simulink model "ps_mass_balance"  (R2025a)
settings: Solver=VariableStepAuto  StartTime=0.0  StopTime=10.0  RelTol=1e-3
libraries: nesl_utility x10, fl_lib x3
settings Model: Creator=degoede  LastModifiedBy=degoede

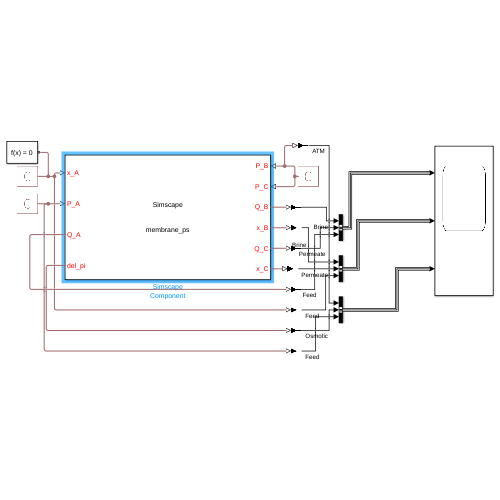
[thumbnail: Simulink's stored preview of the top-level diagram]
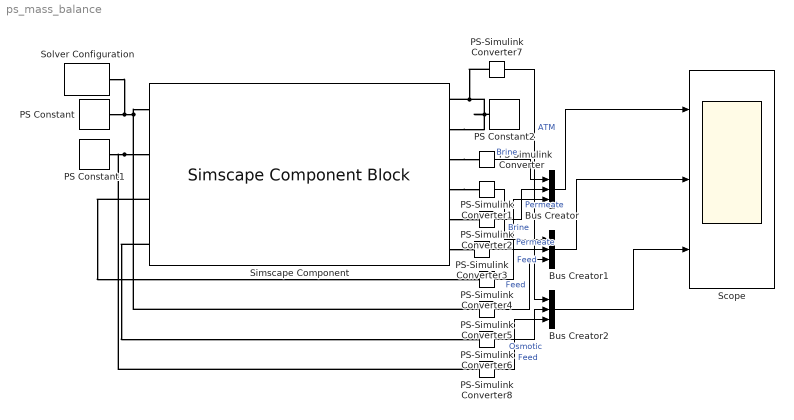
== system ps_mass_balance ==
  Bus Creator : BusCreator  Inputs=3
  Bus Creator1 : BusCreator  Inputs=3
  Bus Creator2 : BusCreator  Inputs=3
  PS Constant : fl_lib/Physical Signals/Sources/PS Constant  constant=36 kg/m^3
  PS Constant1 : fl_lib/Physical Signals/Sources/PS Constant  constant=6e6 Pa
  PS Constant2 : fl_lib/Physical Signals/Sources/PS Constant  constant=1 atm
  PS-Simulink Converter{,1..8} (9 alike) : nesl_utility/PS-Simulink Converter  PhysicalDomain=network_engine_domain  SubClassName=ps_output  LeftPortType=input  RightPortType=output  PseudoPeriodic=off  Frequencies=[]  VectorFormat=inherit  Unit=inherit  AffineConversion=off
  Scope : Scope  NumInputPorts=3
      settings: ActiveDisplayString=3  ActiveDisplayYMinimum=-749998.875  ActiveDisplayYMaximum=6.7499998750000009E+6  YLabel=Pressure [Pa]
  Simscape Component : SimscapeComponentBlock  SourceFile=customization.inouttest.membrane_ps  ComponentPath=customization.inouttest.membrane_ps  ComponentVariants="[\"customization.inouttest.membrane_ps\"]"  ComponentVariantNames="[\"membrane_ps\"]"  ClassName=membrane_ps  SchemaVersion=1  A_w=2.57e-12 m^3/(N*s)  B_s=2.30e-8 m/s  A_m=35*200 m^2  T=273 K  R=8.314 J/(K*mol)  i=2  M=58.44 g/mol  rho_w=1000 kg/m^3  R_B=62e6 Pa*s/m^3
      settings: CopyFcn=simscape.sscblock.internal.componentBlockCallback(gcbh,'COPY')  PreCopyFcn=simscape.sscblock.internal.componentBlockCallback(gcbh,'PRECOPY')  PreDeleteFcn=simscape.sscblock.internal.componentBlockCallback(gcbh,'PREDELETE')  InternalSimscapePortConfiguration="{\"Bottom\":[],\"Left\":[{\"id\":\"x_A\",\"label\":\"x_A\",\"type\":\"input\"},{\"id\":\"P_A\",\"label\":\"P_A\",\"type\":\"input\"},{\"id\":\"Q_A\",\"label\":\"Q_A\",\"type\":\"output\"},{\"id\":\"del_pi\",\"label\":\"del_pi\",\"type\":\"output\"}],\"Right\":[{\"id\":\"P_B\",\"label\":\"P_B\",\"type\":\"input\"},{\"id\":\"P_C\",\"label\":\"P_C\",\"type\":\"input\"},{\"id\":\"Q_B\",\"label\":\"Q_B\",\"type\":\"output\"},{\"id\":\"x_B\",\"label\":\"x_B\",\"type\":\"output\"},{\"id\":\"Q_C\",\"label\":\"Q_C\",\"type\":\"output\"},{\"id\":\"x_C\",\"label\":\"x_C\",\"type\":\"output\"}],\"Top\":[]}"
      mask Type: Membrane (PS)
  Solver Configuration : nesl_utility/Solver Configuration  PhysicalDomain=network_engine_domain  SubClassName=solver  LeftPortType=input  RightPortType=generic  Tones=[]  Harmonics=[]  SimulateNoise=off  Profile=off  UseLocalSampling=off  EnableSwitchedLinearOptims=on  FrequencyDomain=off  UseCCode=off  RelTol=0.001  AbsTol=0.001  MinStep=1e-09  ToWorkspace=off  RevertToSquareIcSolve=off  NumHomotopyIterations=100  PhasorMode=off  PhasorModeNumHarmonics=1  ConsistencySolver=NEWTON_XTOL_AFTER_FTOL  IndexReductionMethod=DerivativeReplacement  DoDC=off  ResidualTolerance=1e-09  ConsistencyTolSource=GLOBAL  ConsistencyAbsTol=0.001  ConsistencyRelTol=0.001  ConsistencyTolFactor=0.001  UseLocalSolver=off  LocalSolverChoice=NE_BACKWARD_EULER_ADVANCER  ResolveIndetEquations=on  FunctionEvalNumThread=1  LocalSolverSampleTime=0.001  DoFixedCost=off  MaxNonlinIter=3  MaxModeIter=2  ComputeImpulses=off  ImpulseIterations=2  LinearAlgebra=auto  LinearAlgebraNumThread=0  EquationFormulation=NE_TIME_EF  DelaysMemoryBudget=1024  AutomaticFiltering=on  FilteringTimeConstant=0.001  PartitionStorageMethod=AS_NEEDED  PartitionMemoryBudget=1024  PartitionMethod=ROBUST  MultibodyUseLocalSolver=off  MultibodyLocalSolverChoice=ODE1  MultibodyLocalSolverSampleTime=0.001
  wires:
  PS-Simulink Converter4/1 -> Bus Creator/3  "Feed"
  PS-Simulink Converter/1 -> Bus Creator/1  "Brine"
  PS-Simulink Converter2/1 -> Bus Creator/2  "Permeate"
  PS-Simulink Converter1/1 -> Bus Creator1/1  "Brine"
  PS-Simulink Converter3/1 -> Bus Creator1/2  "Permeate"
  Bus Creator/1 -> Scope/1
  Bus Creator1/1 -> Scope/2
  PS-Simulink Converter5/1 -> Bus Creator1/3  "Feed"
  PS-Simulink Converter6/1 -> Bus Creator2/2  "Osmotic"
  PS-Simulink Converter7/1 -> Bus Creator2/1  "ATM"
  PS-Simulink Converter8/1 -> Bus Creator2/3  "Feed"
  Bus Creator2/1 -> Scope/3
  connections:
  PS Constant/RConn1 -- Solver Configuration/RConn1 -- PS-Simulink Converter5/LConn1 -- Simscape Component/LConn1
  PS Constant1/RConn1 -- Simscape Component/LConn2 -- PS-Simulink Converter8/LConn1
  PS Constant2/RConn1 -- PS-Simulink Converter7/LConn1 -- Simscape Component/RConn1 -- Simscape Component/RConn2
  Simscape Component/RConn6 -- PS-Simulink Converter3/LConn1
  Simscape Component/RConn5 -- PS-Simulink Converter2/LConn1
  Simscape Component/RConn4 -- PS-Simulink Converter1/LConn1
  Simscape Component/RConn3 -- PS-Simulink Converter/LConn1
  Simscape Component/LConn3 -- PS-Simulink Converter4/LConn1
  Simscape Component/LConn4 -- PS-Simulink Converter6/LConn1
